simulink model "elevatorMod"  (R2020a)
settings: Solver=VariableStepAuto  StartTime=0.0  StopTime=inf  RelTol=1e-3
PreLoadFcn:
  | slplc.api.loadDataTypes;
undefined symbols (not defined in the file): BOOL, DINT, INT, slplc
libraries: simulink x1
(part 16 of 39)

== system elevatorMod/PLCControllerSuite/__Logic/Task/Program/__Logic/SUB/RungOutOverride ==
  In1 : Inport
  AND : Logic  AllPortsSameDT=off  OutDataTypeStr=boolean
  BlockEnableRead : Subsystem  DisableCoverage=on  TreatAsAtomicUnit=on  mask{PLCLabelTag=_Block_Enable, PLCBlockType=BlockEnableRead}
      mask prompts: PLCLabelTag "Label Tag:"
      mask init:
      | block = gcb;
      | maskObj = Simulink.Mask.get(block);
      | maskObj.Display = sprintf('disp(''%s'');', PLCLabelTag);
      mask Help: web([docroot '/plccoder/ref/blockenableread' '.html']);
      mask DialogControl PLCBlockTitle Prompt: Block Enable Read
      mask Display: disp('_Block_Enable');
  VariableWriteEnableWrite : Subsystem  DisableCoverage=on  TreatAsAtomicUnit=on  mask{PLCLabelTag=_Variable_Write_Enable, PLCBlockType=VariableWriteEnableWrite}
      mask prompts: PLCLabelTag "Label Tag:"
      mask init:
      | block = gcb;
      | maskObj = Simulink.Mask.get(block);
      | maskObj.Display = sprintf('disp(''%s'');', PLCLabelTag);
      mask Help: web([docroot '/plccoder/ref/variablewriteenablewrite' '.html']);
      mask DialogControl PLCBlockTitle Prompt: Variable Write_Enable_Write
      mask Display: disp('_Variable_Write_Enable');
  Out1 : Outport  VectorParamsAs1DForOutWhenUnconnected=off
  wires:
  AND/1 -> VariableWriteEnableWrite/1(In1), Out1/1
  BlockEnableRead/1(Out1) -> AND/1
  In1/1 -> AND/2

== system elevatorMod/PLCControllerSuite/__Logic/Task/Program/__Logic/TON/BlockEnableRead ==
  __CoreLabelRead : Subsystem  Tag=CoreVarReadBlock  DisableCoverage=on  TreatAsAtomicUnit=on  mask{PLCBlockType=CoreLabelRead}
      mask init:
      | slplc.callbacks.initRoutineLabelRead(gcb);
      mask Help: web([docroot '/plccoder/ref/__corelabelread' '.html']);
      mask DialogControl PLCBlockTitle Prompt: Core Label Read
  Out1 : Outport  VectorParamsAs1DForOutWhenUnconnected=off
  wires:
  __CoreLabelRead/1(Out1) -> Out1/1

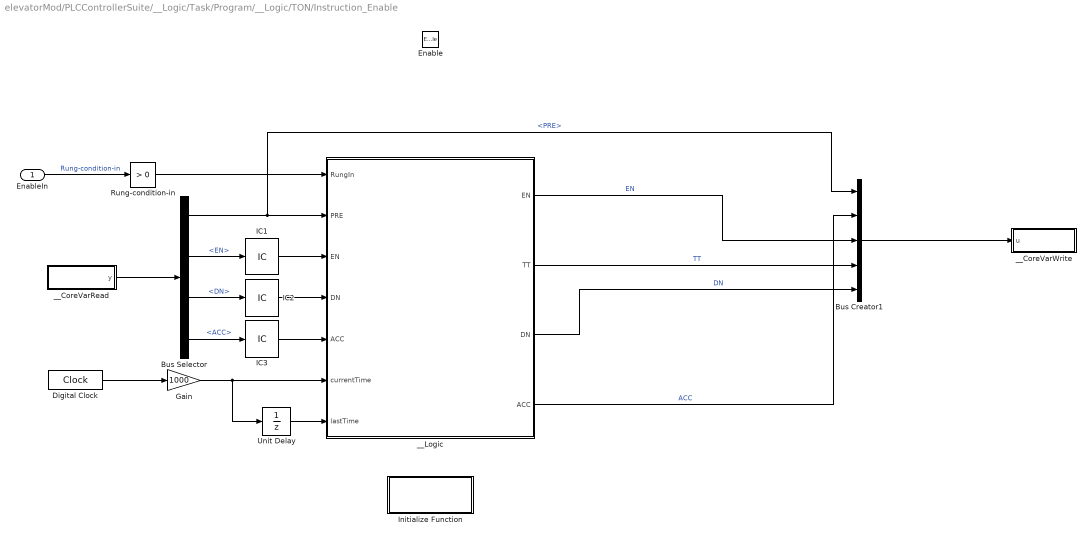
== system elevatorMod/PLCControllerSuite/__Logic/Task/Program/__Logic/TON/Instruction_Enable ==
  EnableIn : Inport
  Enable : EnablePort
  Bus Creator1 : BusCreator  Inputs=5  OutDataTypeStr=Bus: TIMER  NonVirtualBus=on
  Bus Selector : BusSelector  OutputSignals=PRE,EN,DN,ACC
  Digital Clock : DigitalClock  SampleTime=PLCTimerSampleTime
  Gain : Gain  Gain=1000
  IC1 : InitialCondition  Value=false
  IC2 : InitialCondition  Value=false
  IC3 : InitialCondition  Value=0
  Initialize Function : Subsystem  TreatAsAtomicUnit=on
  Rung-condition-in : simulink/Logic and Bit Operations/Compare To Zero  relop=>  OutDataTypeStr=boolean
  Unit Delay : UnitDelay  SampleTime=-1  HasFrameUpgradeWarning=on
  __CoreVarRead : Subsystem  Tag=CoreVarReadBlock  DisableCoverage=on  TreatAsAtomicUnit=on  mask{PLCBlockType=CoreVarRead}
      mask init:
      | slplc.callbacks.initCoreVariable(gcb, 'read');
      mask Help: web([docroot '/plccoder/ref/__corevarread' '.html']);
      mask DialogControl PLCBlockTitle Prompt: Core Variable Read
  __CoreVarWrite : Subsystem  Tag=CoreVarWriteBlock  DisableCoverage=on  TreatAsAtomicUnit=on  mask{PLCBlockType=CoreVarWrite}
      mask init:
      | slplc.callbacks.initCoreVariable(gcb, 'write');
      mask Help: web([docroot '/plccoder/ref/__corevarwrite' '.html']);
      mask DialogControl PLCBlockTitle Prompt: Core Variable Write
  __Logic : MATLAB Function  Priority=12  DisableCoverage=on
  wires:
  IC3/1 -> __Logic/5("ACC ")
  IC2/1 -> __Logic/4("DN ")
  IC1/1 -> __Logic/3("EN ")
  Rung-condition-in/1 -> __Logic/1(RungIn)
  Bus Selector/2 -> IC1/1  "<EN>"
  Gain/1 -> __Logic/6(currentTime), Unit Delay/1
  Bus Selector/3 -> IC2/1  "<DN>"
  __CoreVarRead/1(y) -> Bus Selector/1
  Unit Delay/1 -> __Logic/7(lastTime)
  Bus Creator1/1 -> __CoreVarWrite/1(u)
  __Logic/4(ACC) -> Bus Creator1/2  "ACC"
  __Logic/3(DN) -> Bus Creator1/5  "DN"
  Digital Clock/1 -> Gain/1
  EnableIn/1 -> Rung-condition-in/1  "Rung-condition-in"
  Bus Selector/1 -> Bus Creator1/1, __Logic/2(PRE)  "<PRE>"
  __Logic/2(TT) -> Bus Creator1/4  "TT"
  Bus Selector/4 -> IC3/1  "<ACC>"
  __Logic/1(EN) -> Bus Creator1/3  "EN"

== system elevatorMod/PLCControllerSuite/__Logic/Task/Program/__Logic/TON/RungInOverride ==
  In1 : Inport
  AND : Logic  AllPortsSameDT=off  OutDataTypeStr=boolean
  ForceRungInFalseRead : Subsystem  DisableCoverage=on  TreatAsAtomicUnit=on  mask{PLCLabelTag=_Force_RungIn_False, PLCBlockType=ForceRungInFalseRead}
      mask prompts: PLCLabelTag "Label Tag:"
      mask init:
      | block = gcb;
      | maskObj = Simulink.Mask.get(block);
      | maskObj.Display = sprintf('disp(''%s'');', PLCLabelTag);
      mask Help: web([docroot '/plccoder/ref/forcerunginfalseread' '.html']);
      mask DialogControl PLCBlockTitle Prompt: Force Rung-In False Read
      mask Display: disp('_Force_RungIn_False');
  NOT : Logic  Operator=NOT  IconShape=distinctive  AllPortsSameDT=off  OutDataTypeStr=boolean
  Out1 : Outport  VectorParamsAs1DForOutWhenUnconnected=off
  wires:
  AND/1 -> Out1/1
  In1/1 -> AND/2
  ForceRungInFalseRead/1(Out1) -> NOT/1
  NOT/1 -> AND/1

== system elevatorMod/PLCControllerSuite/__Logic/Task/Program/__Logic/TON/__CoreVarRead ==
  DataRead : DataStoreRead  DataStoreName=xxx_PLC_VAR_T
  y : Outport  VectorParamsAs1DForOutWhenUnconnected=off
  wires:
  DataRead/1 -> y/1

== system elevatorMod/PLCControllerSuite/__Logic/Task/Program/__Logic/Variable Read/__CoreVarRead ==
  DataRead : DataStoreRead  DataStoreName=xxx_PLC_VAR_VARVEL
  y : Outport  VectorParamsAs1DForOutWhenUnconnected=off
  wires:
  DataRead/1 -> y/1

== system elevatorMod/PLCControllerSuite/__Logic/Task/Program/__Logic/Variable Read1/__CoreVarRead ==
  DataRead : DataStoreRead  DataStoreName=xxx_PLC_VAR_Floor_1
  y : Outport  VectorParamsAs1DForOutWhenUnconnected=off
  wires:
  DataRead/1 -> y/1

== system elevatorMod/PLCControllerSuite/__Logic/Task/Program/__Logic/Variable Read10/__CoreVarRead ==
  DataRead : DataStoreRead  DataStoreName=xxx_PLC_VAR_VARVEL
  y : Outport  VectorParamsAs1DForOutWhenUnconnected=off
  wires:
  DataRead/1 -> y/1

== system elevatorMod/PLCControllerSuite/__Logic/Task/Program/__Logic/Variable Read11/__CoreVarRead ==
  DataRead : DataStoreRead  DataStoreName=xxx_PLC_VAR_VARVEL
  y : Outport  VectorParamsAs1DForOutWhenUnconnected=off
  wires:
  DataRead/1 -> y/1

== system elevatorMod/PLCControllerSuite/__Logic/Task/Program/__Logic/Variable Read12/__CoreVarRead ==
  DataRead : DataStoreRead  DataStoreName=xxx_PLC_VAR_VARVEL
  y : Outport  VectorParamsAs1DForOutWhenUnconnected=off
  wires:
  DataRead/1 -> y/1

== system elevatorMod/PLCControllerSuite/__Logic/Task/Program/__Logic/Variable Read13/__CoreVarRead ==
  DataRead : DataStoreRead  DataStoreName=xxx_PLC_VAR_VARVEL
  y : Outport  VectorParamsAs1DForOutWhenUnconnected=off
  wires:
  DataRead/1 -> y/1

== system elevatorMod/PLCControllerSuite/__Logic/Task/Program/__Logic/Variable Read14/__CoreVarRead ==
  DataRead : DataStoreRead  DataStoreName=xxx_PLC_VAR_VARVEL
  y : Outport  VectorParamsAs1DForOutWhenUnconnected=off
  wires:
  DataRead/1 -> y/1

== system elevatorMod/PLCControllerSuite/__Logic/Task/Program/__Logic/Variable Read15/__CoreVarRead ==
  DataRead : DataStoreRead  DataStoreName=xxx_PLC_VAR_VARVEL
  y : Outport  VectorParamsAs1DForOutWhenUnconnected=off
  wires:
  DataRead/1 -> y/1

== system elevatorMod/PLCControllerSuite/__Logic/Task/Program/__Logic/Variable Read16/__CoreVarRead ==
  DataRead : DataStoreRead  DataStoreName=xxx_PLC_VAR_Current_floor
  y : Outport  VectorParamsAs1DForOutWhenUnconnected=off
  wires:
  DataRead/1 -> y/1

== system elevatorMod/PLCControllerSuite/__Logic/Task/Program/__Logic/Variable Read2/__CoreVarRead ==
  DataRead : DataStoreRead  DataStoreName=xxx_PLC_VAR_Floor_2
  y : Outport  VectorParamsAs1DForOutWhenUnconnected=off
  wires:
  DataRead/1 -> y/1

== system elevatorMod/PLCControllerSuite/__Logic/Task/Program/__Logic/Variable Read3/__CoreVarRead ==
  DataRead : DataStoreRead  DataStoreName=xxx_PLC_VAR_Floor_3
  y : Outport  VectorParamsAs1DForOutWhenUnconnected=off
  wires:
  DataRead/1 -> y/1

== system elevatorMod/PLCControllerSuite/__Logic/Task/Program/__Logic/Variable Read4/__CoreVarRead ==
  DataRead : DataStoreRead  DataStoreName=xxx_PLC_VAR_Floor_1
  y : Outport  VectorParamsAs1DForOutWhenUnconnected=off
  wires:
  DataRead/1 -> y/1

== system elevatorMod/PLCControllerSuite/__Logic/Task/Program/__Logic/Variable Read5/__CoreVarRead ==
  DataRead : DataStoreRead  DataStoreName=xxx_PLC_VAR_Current_floor
  y : Outport  VectorParamsAs1DForOutWhenUnconnected=off
  wires:
  DataRead/1 -> y/1

== system elevatorMod/PLCControllerSuite/__Logic/Task/Program/__Logic/Variable Read6/__CoreVarRead ==
  DataRead : DataStoreRead  DataStoreName=xxx_PLC_VAR_Floor_2
  y : Outport  VectorParamsAs1DForOutWhenUnconnected=off
  wires:
  DataRead/1 -> y/1

== system elevatorMod/PLCControllerSuite/__Logic/Task/Program/__Logic/Variable Read7/__CoreVarRead ==
  DataRead : DataStoreRead  DataStoreName=xxx_PLC_VAR_Current_floor
  y : Outport  VectorParamsAs1DForOutWhenUnconnected=off
  wires:
  DataRead/1 -> y/1

== system elevatorMod/PLCControllerSuite/__Logic/Task/Program/__Logic/Variable Read8/__CoreVarRead ==
  DataRead : DataStoreRead  DataStoreName=xxx_PLC_VAR_Floor_3
  y : Outport  VectorParamsAs1DForOutWhenUnconnected=off
  wires:
  DataRead/1 -> y/1

== system elevatorMod/PLCControllerSuite/__Logic/Task/Program/__Logic/Variable Read9/__CoreVarRead ==
  DataRead : DataStoreRead  DataStoreName=xxx_PLC_VAR_Current_floor
  y : Outport  VectorParamsAs1DForOutWhenUnconnected=off
  wires:
  DataRead/1 -> y/1

== system elevatorMod/PLCControllerSuite/__Logic/Task/Program/__Logic/Variable Write1/VariableWriteEnableRead ==
  __CoreLabelRead : Subsystem  Tag=CoreVarReadBlock  DisableCoverage=on  TreatAsAtomicUnit=on  mask{PLCBlockType=CoreLabelRead}
      mask init:
      | slplc.callbacks.initRoutineLabelRead(gcb);
      mask Help: web([docroot '/plccoder/ref/__corelabelread' '.html']);
      mask DialogControl PLCBlockTitle Prompt: Core Label Read
  Out1 : Outport  VectorParamsAs1DForOutWhenUnconnected=off
  wires:
  __CoreLabelRead/1(Out1) -> Out1/1

== system elevatorMod/PLCControllerSuite/__Logic/Task/Program/__Logic/Variable Write1/__CoreVarRead ==
  DataRead : DataStoreRead  DataStoreName=xxx_PLC_VAR_Current_floor
  y : Outport  VectorParamsAs1DForOutWhenUnconnected=off
  wires:
  DataRead/1 -> y/1

== system elevatorMod/PLCControllerSuite/__Logic/Task/Program/__Logic/Variable Write1/__Enable ==
  VarIn : Inport
  Enable : EnablePort
  __CoreVarWrite : Subsystem  Tag=CoreVarWriteBlock  DisableCoverage=on  TreatAsAtomicUnit=on  mask{PLCBlockType=CoreVarWrite}
      mask init:
      | slplc.callbacks.initCoreVariable(gcb, 'write');
      mask Help: web([docroot '/plccoder/ref/__corevarwrite' '.html']);
      mask DialogControl PLCBlockTitle Prompt: Core Variable Write
  wires:
  VarIn/1 -> __CoreVarWrite/1(u)

== system elevatorMod/PLCControllerSuite/__Logic/Task/Program/__Logic/Variable Write2/VariableWriteEnableRead ==
  __CoreLabelRead : Subsystem  Tag=CoreVarReadBlock  DisableCoverage=on  TreatAsAtomicUnit=on  mask{PLCBlockType=CoreLabelRead}
      mask init:
      | slplc.callbacks.initRoutineLabelRead(gcb);
      mask Help: web([docroot '/plccoder/ref/__corelabelread' '.html']);
      mask DialogControl PLCBlockTitle Prompt: Core Label Read
  Out1 : Outport  VectorParamsAs1DForOutWhenUnconnected=off
  wires:
  __CoreLabelRead/1(Out1) -> Out1/1

== system elevatorMod/PLCControllerSuite/__Logic/Task/Program/__Logic/Variable Write2/__CoreVarRead ==
  DataRead : DataStoreRead  DataStoreName=xxx_PLC_VAR_Current_floor
  y : Outport  VectorParamsAs1DForOutWhenUnconnected=off
  wires:
  DataRead/1 -> y/1

== system elevatorMod/PLCControllerSuite/__Logic/Task/Program/__Logic/Variable Write2/__Enable ==
  VarIn : Inport
  Enable : EnablePort
  __CoreVarWrite : Subsystem  Tag=CoreVarWriteBlock  DisableCoverage=on  TreatAsAtomicUnit=on  mask{PLCBlockType=CoreVarWrite}
      mask init:
      | slplc.callbacks.initCoreVariable(gcb, 'write');
      mask Help: web([docroot '/plccoder/ref/__corevarwrite' '.html']);
      mask DialogControl PLCBlockTitle Prompt: Core Variable Write
  wires:
  VarIn/1 -> __CoreVarWrite/1(u)

== system elevatorMod/PLCControllerSuite/__Logic/Task/Program/__Logic/Variable Write3/VariableWriteEnableRead ==
  __CoreLabelRead : Subsystem  Tag=CoreVarReadBlock  DisableCoverage=on  TreatAsAtomicUnit=on  mask{PLCBlockType=CoreLabelRead}
      mask init:
      | slplc.callbacks.initRoutineLabelRead(gcb);
      mask Help: web([docroot '/plccoder/ref/__corelabelread' '.html']);
      mask DialogControl PLCBlockTitle Prompt: Core Label Read
  Out1 : Outport  VectorParamsAs1DForOutWhenUnconnected=off
  wires:
  __CoreLabelRead/1(Out1) -> Out1/1

== system elevatorMod/PLCControllerSuite/__Logic/Task/Program/__Logic/Variable Write3/__CoreVarRead ==
  DataRead : DataStoreRead  DataStoreName=xxx_PLC_VAR_Current_floor
  y : Outport  VectorParamsAs1DForOutWhenUnconnected=off
  wires:
  DataRead/1 -> y/1

== system elevatorMod/PLCControllerSuite/__Logic/Task/Program/__Logic/Variable Write3/__Enable ==
  VarIn : Inport
  Enable : EnablePort
  __CoreVarWrite : Subsystem  Tag=CoreVarWriteBlock  DisableCoverage=on  TreatAsAtomicUnit=on  mask{PLCBlockType=CoreVarWrite}
      mask init:
      | slplc.callbacks.initCoreVariable(gcb, 'write');
      mask Help: web([docroot '/plccoder/ref/__corevarwrite' '.html']);
      mask DialogControl PLCBlockTitle Prompt: Core Variable Write
  wires:
  VarIn/1 -> __CoreVarWrite/1(u)

== system elevatorMod/PLCControllerSuite/__Logic/Task/Program/__Logic/Variable Write4/VariableWriteEnableRead ==
  __CoreLabelRead : Subsystem  Tag=CoreVarReadBlock  DisableCoverage=on  TreatAsAtomicUnit=on  mask{PLCBlockType=CoreLabelRead}
      mask init:
      | slplc.callbacks.initRoutineLabelRead(gcb);
      mask Help: web([docroot '/plccoder/ref/__corelabelread' '.html']);
      mask DialogControl PLCBlockTitle Prompt: Core Label Read
  Out1 : Outport  VectorParamsAs1DForOutWhenUnconnected=off
  wires:
  __CoreLabelRead/1(Out1) -> Out1/1

== system elevatorMod/PLCControllerSuite/__Logic/Task/Program/__Logic/Variable Write4/__CoreVarRead ==
  DataRead : DataStoreRead  DataStoreName=xxx_PLC_VAR_VARVEL
  y : Outport  VectorParamsAs1DForOutWhenUnconnected=off
  wires:
  DataRead/1 -> y/1

== system elevatorMod/PLCControllerSuite/__Logic/Task/Program/__Logic/Variable Write4/__Enable ==
  VarIn : Inport
  Enable : EnablePort
  __CoreVarWrite : Subsystem  Tag=CoreVarWriteBlock  DisableCoverage=on  TreatAsAtomicUnit=on  mask{PLCBlockType=CoreVarWrite}
      mask init:
      | slplc.callbacks.initCoreVariable(gcb, 'write');
      mask Help: web([docroot '/plccoder/ref/__corevarwrite' '.html']);
      mask DialogControl PLCBlockTitle Prompt: Core Variable Write
  wires:
  VarIn/1 -> __CoreVarWrite/1(u)

== system elevatorMod/PLCControllerSuite/__Logic/Task/Program/__Logic/Variable Write5/VariableWriteEnableRead ==
  __CoreLabelRead : Subsystem  Tag=CoreVarReadBlock  DisableCoverage=on  TreatAsAtomicUnit=on  mask{PLCBlockType=CoreLabelRead}
      mask init:
      | slplc.callbacks.initRoutineLabelRead(gcb);
      mask Help: web([docroot '/plccoder/ref/__corelabelread' '.html']);
      mask DialogControl PLCBlockTitle Prompt: Core Label Read
  Out1 : Outport  VectorParamsAs1DForOutWhenUnconnected=off
  wires:
  __CoreLabelRead/1(Out1) -> Out1/1

== system elevatorMod/PLCControllerSuite/__Logic/Task/Program/__Logic/Variable Write5/__CoreVarRead ==
  DataRead : DataStoreRead  DataStoreName=xxx_PLC_VAR_VARVEL
  y : Outport  VectorParamsAs1DForOutWhenUnconnected=off
  wires:
  DataRead/1 -> y/1

== system elevatorMod/PLCControllerSuite/__Logic/Task/Program/__Logic/Variable Write5/__Enable ==
  VarIn : Inport
  Enable : EnablePort
  __CoreVarWrite : Subsystem  Tag=CoreVarWriteBlock  DisableCoverage=on  TreatAsAtomicUnit=on  mask{PLCBlockType=CoreVarWrite}
      mask init:
      | slplc.callbacks.initCoreVariable(gcb, 'write');
      mask Help: web([docroot '/plccoder/ref/__corevarwrite' '.html']);
      mask DialogControl PLCBlockTitle Prompt: Core Variable Write
  wires:
  VarIn/1 -> __CoreVarWrite/1(u)

== system elevatorMod/PLCControllerSuite/__Logic/Task/Program/__Logic/Variable Write6/VariableWriteEnableRead ==
  __CoreLabelRead : Subsystem  Tag=CoreVarReadBlock  DisableCoverage=on  TreatAsAtomicUnit=on  mask{PLCBlockType=CoreLabelRead}
      mask init:
      | slplc.callbacks.initRoutineLabelRead(gcb);
      mask Help: web([docroot '/plccoder/ref/__corelabelread' '.html']);
      mask DialogControl PLCBlockTitle Prompt: Core Label Read
  Out1 : Outport  VectorParamsAs1DForOutWhenUnconnected=off
  wires:
  __CoreLabelRead/1(Out1) -> Out1/1

== system elevatorMod/PLCControllerSuite/__Logic/Task/Program/__Logic/Variable Write6/__CoreVarRead ==
  DataRead : DataStoreRead  DataStoreName=xxx_PLC_VAR_VARVEL
  y : Outport  VectorParamsAs1DForOutWhenUnconnected=off
  wires:
  DataRead/1 -> y/1

== system elevatorMod/PLCControllerSuite/__Logic/Task/Program/__Logic/Variable Write6/__Enable ==
  VarIn : Inport
  Enable : EnablePort
  __CoreVarWrite : Subsystem  Tag=CoreVarWriteBlock  DisableCoverage=on  TreatAsAtomicUnit=on  mask{PLCBlockType=CoreVarWrite}
      mask init:
      | slplc.callbacks.initCoreVariable(gcb, 'write');
      mask Help: web([docroot '/plccoder/ref/__corevarwrite' '.html']);
      mask DialogControl PLCBlockTitle Prompt: Core Variable Write
  wires:
  VarIn/1 -> __CoreVarWrite/1(u)

== system elevatorMod/PLCControllerSuite/__Logic/Task/Program/__Logic/Variable Write7/VariableWriteEnableRead ==
  __CoreLabelRead : Subsystem  Tag=CoreVarReadBlock  DisableCoverage=on  TreatAsAtomicUnit=on  mask{PLCBlockType=CoreLabelRead}
      mask init:
      | slplc.callbacks.initRoutineLabelRead(gcb);
      mask Help: web([docroot '/plccoder/ref/__corelabelread' '.html']);
      mask DialogControl PLCBlockTitle Prompt: Core Label Read
  Out1 : Outport  VectorParamsAs1DForOutWhenUnconnected=off
  wires:
  __CoreLabelRead/1(Out1) -> Out1/1

== system elevatorMod/PLCControllerSuite/__Logic/Task/Program/__Logic/Variable Write7/__CoreVarRead ==
  DataRead : DataStoreRead  DataStoreName=xxx_PLC_VAR_VELOUT
  y : Outport  VectorParamsAs1DForOutWhenUnconnected=off
  wires:
  DataRead/1 -> y/1

== system elevatorMod/PLCControllerSuite/__Logic/Task/Program/__Logic/Variable Write7/__Enable ==
  VarIn : Inport
  Enable : EnablePort
  __CoreVarWrite : Subsystem  Tag=CoreVarWriteBlock  DisableCoverage=on  TreatAsAtomicUnit=on  mask{PLCBlockType=CoreVarWrite}
      mask init:
      | slplc.callbacks.initCoreVariable(gcb, 'write');
      mask Help: web([docroot '/plccoder/ref/__corevarwrite' '.html']);
      mask DialogControl PLCBlockTitle Prompt: Core Variable Write
  wires:
  VarIn/1 -> __CoreVarWrite/1(u)

== system elevatorMod/PLCControllerSuite/__Logic/Task/Program/__Logic/Variable Write8/VariableWriteEnableRead ==
  __CoreLabelRead : Subsystem  Tag=CoreVarReadBlock  DisableCoverage=on  TreatAsAtomicUnit=on  mask{PLCBlockType=CoreLabelRead}
      mask init:
      | slplc.callbacks.initRoutineLabelRead(gcb);
      mask Help: web([docroot '/plccoder/ref/__corelabelread' '.html']);
      mask DialogControl PLCBlockTitle Prompt: Core Label Read
  Out1 : Outport  VectorParamsAs1DForOutWhenUnconnected=off
  wires:
  __CoreLabelRead/1(Out1) -> Out1/1

== system elevatorMod/PLCControllerSuite/__Logic/Task/Program/__Logic/Variable Write8/__CoreVarRead ==
  DataRead : DataStoreRead  DataStoreName=xxx_PLC_VAR_FLOOROUT
  y : Outport  VectorParamsAs1DForOutWhenUnconnected=off
  wires:
  DataRead/1 -> y/1

== system elevatorMod/PLCControllerSuite/__Logic/Task/Program/__Logic/Variable Write8/__Enable ==
  VarIn : Inport
  Enable : EnablePort
  __CoreVarWrite : Subsystem  Tag=CoreVarWriteBlock  DisableCoverage=on  TreatAsAtomicUnit=on  mask{PLCBlockType=CoreVarWrite}
      mask init:
      | slplc.callbacks.initCoreVariable(gcb, 'write');
      mask Help: web([docroot '/plccoder/ref/__corevarwrite' '.html']);
      mask DialogControl PLCBlockTitle Prompt: Core Variable Write
  wires:
  VarIn/1 -> __CoreVarWrite/1(u)

== system elevatorMod/PLCControllerSuite/__Logic/Task/Program/__Logic/XIC/BlockEnableRead ==
  __CoreLabelRead : Subsystem  Tag=CoreVarReadBlock  DisableCoverage=on  TreatAsAtomicUnit=on  mask{PLCBlockType=CoreLabelRead}
      mask init:
      | slplc.callbacks.initRoutineLabelRead(gcb);
      mask Help: web([docroot '/plccoder/ref/__corelabelread' '.html']);
      mask DialogControl PLCBlockTitle Prompt: Core Label Read
  Out1 : Outport  VectorParamsAs1DForOutWhenUnconnected=off
  wires:
  __CoreLabelRead/1(Out1) -> Out1/1

== system elevatorMod/PLCControllerSuite/__Logic/Task/Program/__Logic/XIC/Instruction_Enable ==
  Rung-condition-in : Inport  OutDataTypeStr=BOOL
  Enable : EnablePort
  Logical Operator : Logic  OutDataTypeStr=BOOL
  __CoreVarRead : Subsystem  Tag=CoreVarReadBlock  DisableCoverage=on  TreatAsAtomicUnit=on  mask{PLCBlockType=CoreVarRead}
      mask init:
      | slplc.callbacks.initCoreVariable(gcb, 'read');
      mask Help: web([docroot '/plccoder/ref/__corevarread' '.html']);
      mask DialogControl PLCBlockTitle Prompt: Core Variable Read
  Rung-condition-out : Outport  VectorParamsAs1DForOutWhenUnconnected=off
  wires:
  __CoreVarRead/1(y) -> Logical Operator/2  "DataBit"
  Logical Operator/1 -> Rung-condition-out/1  "Rung-condition-out"
  Rung-condition-in/1 -> Logical Operator/1  "Rung-condition-in"

== system elevatorMod/PLCControllerSuite/__Logic/Task/Program/__Logic/XIC/RungInOverride ==
  In1 : Inport
  AND : Logic  AllPortsSameDT=off  OutDataTypeStr=boolean
  ForceRungInFalseRead : Subsystem  DisableCoverage=on  TreatAsAtomicUnit=on  mask{PLCLabelTag=_Force_RungIn_False, PLCBlockType=ForceRungInFalseRead}
      mask prompts: PLCLabelTag "Label Tag:"
      mask init:
      | block = gcb;
      | maskObj = Simulink.Mask.get(block);
      | maskObj.Display = sprintf('disp(''%s'');', PLCLabelTag);
      mask Help: web([docroot '/plccoder/ref/forcerunginfalseread' '.html']);
      mask DialogControl PLCBlockTitle Prompt: Force Rung-In False Read
      mask Display: disp('_Force_RungIn_False');
  NOT : Logic  Operator=NOT  IconShape=distinctive  AllPortsSameDT=off  OutDataTypeStr=boolean
  Out1 : Outport  VectorParamsAs1DForOutWhenUnconnected=off
  wires:
  NOT/1 -> AND/1
  ForceRungInFalseRead/1(Out1) -> NOT/1
  In1/1 -> AND/2
  AND/1 -> Out1/1

== system elevatorMod/PLCControllerSuite/__Logic/Task/Program/__Logic/XIC/__CoreVarRead ==
  DataRead : DataStoreRead  DataStoreName=xxx_PLC_VAR_Start
  y : Outport  VectorParamsAs1DForOutWhenUnconnected=off
  wires:
  DataRead/1 -> y/1

== system elevatorMod/PLCControllerSuite/__Logic/Task/Program/__Logic/XIC1/BlockEnableRead ==
  __CoreLabelRead : Subsystem  Tag=CoreVarReadBlock  DisableCoverage=on  TreatAsAtomicUnit=on  mask{PLCBlockType=CoreLabelRead}
      mask init:
      | slplc.callbacks.initRoutineLabelRead(gcb);
      mask Help: web([docroot '/plccoder/ref/__corelabelread' '.html']);
      mask DialogControl PLCBlockTitle Prompt: Core Label Read
  Out1 : Outport  VectorParamsAs1DForOutWhenUnconnected=off
  wires:
  __CoreLabelRead/1(Out1) -> Out1/1

== system elevatorMod/PLCControllerSuite/__Logic/Task/Program/__Logic/XIC1/Instruction_Enable ==
  Rung-condition-in : Inport  OutDataTypeStr=BOOL
  Enable : EnablePort
  Logical Operator : Logic  OutDataTypeStr=BOOL
  __CoreVarRead : Subsystem  Tag=CoreVarReadBlock  DisableCoverage=on  TreatAsAtomicUnit=on  mask{PLCBlockType=CoreVarRead}
      mask init:
      | slplc.callbacks.initCoreVariable(gcb, 'read');
      mask Help: web([docroot '/plccoder/ref/__corevarread' '.html']);
      mask DialogControl PLCBlockTitle Prompt: Core Variable Read
  Rung-condition-out : Outport  VectorParamsAs1DForOutWhenUnconnected=off
  wires:
  __CoreVarRead/1(y) -> Logical Operator/2  "DataBit"
  Logical Operator/1 -> Rung-condition-out/1  "Rung-condition-out"
  Rung-condition-in/1 -> Logical Operator/1  "Rung-condition-in"

== system elevatorMod/PLCControllerSuite/__Logic/Task/Program/__Logic/XIC1/RungInOverride ==
  In1 : Inport
  AND : Logic  AllPortsSameDT=off  OutDataTypeStr=boolean
  ForceRungInFalseRead : Subsystem  DisableCoverage=on  TreatAsAtomicUnit=on  mask{PLCLabelTag=_Force_RungIn_False, PLCBlockType=ForceRungInFalseRead}
      mask prompts: PLCLabelTag "Label Tag:"
      mask init:
      | block = gcb;
      | maskObj = Simulink.Mask.get(block);
      | maskObj.Display = sprintf('disp(''%s'');', PLCLabelTag);
      mask Help: web([docroot '/plccoder/ref/forcerunginfalseread' '.html']);
      mask DialogControl PLCBlockTitle Prompt: Force Rung-In False Read
      mask Display: disp('_Force_RungIn_False');
  NOT : Logic  Operator=NOT  IconShape=distinctive  AllPortsSameDT=off  OutDataTypeStr=boolean
  Out1 : Outport  VectorParamsAs1DForOutWhenUnconnected=off
  wires:
  NOT/1 -> AND/1
  ForceRungInFalseRead/1(Out1) -> NOT/1
  In1/1 -> AND/2
  AND/1 -> Out1/1

== system elevatorMod/PLCControllerSuite/__Logic/Task/Program/__Logic/XIC1/__CoreVarRead ==
  DataRead : DataStoreRead  DataStoreName=xxx_PLC_VAR_StartHold
  y : Outport  VectorParamsAs1DForOutWhenUnconnected=off
  wires:
  DataRead/1 -> y/1

== system elevatorMod/PLCControllerSuite/__Logic/Task/Program/__Logic/XIC10/BlockEnableRead ==
  __CoreLabelRead : Subsystem  Tag=CoreVarReadBlock  DisableCoverage=on  TreatAsAtomicUnit=on  mask{PLCBlockType=CoreLabelRead}
      mask init:
      | slplc.callbacks.initRoutineLabelRead(gcb);
      mask Help: web([docroot '/plccoder/ref/__corelabelread' '.html']);
      mask DialogControl PLCBlockTitle Prompt: Core Label Read
  Out1 : Outport  VectorParamsAs1DForOutWhenUnconnected=off
  wires:
  __CoreLabelRead/1(Out1) -> Out1/1

== system elevatorMod/PLCControllerSuite/__Logic/Task/Program/__Logic/XIC10/Instruction_Enable ==
  Rung-condition-in : Inport  OutDataTypeStr=BOOL
  Enable : EnablePort
  Logical Operator : Logic  OutDataTypeStr=BOOL
  __CoreVarRead : Subsystem  Tag=CoreVarReadBlock  DisableCoverage=on  TreatAsAtomicUnit=on  mask{PLCBlockType=CoreVarRead}
      mask init:
      | slplc.callbacks.initCoreVariable(gcb, 'read');
      mask Help: web([docroot '/plccoder/ref/__corevarread' '.html']);
      mask DialogControl PLCBlockTitle Prompt: Core Variable Read
  Rung-condition-out : Outport  VectorParamsAs1DForOutWhenUnconnected=off
  wires:
  Rung-condition-in/1 -> Logical Operator/1  "Rung-condition-in"
  Logical Operator/1 -> Rung-condition-out/1  "Rung-condition-out"
  __CoreVarRead/1(y) -> Logical Operator/2  "DataBit"

== system elevatorMod/PLCControllerSuite/__Logic/Task/Program/__Logic/XIC10/RungInOverride ==
  In1 : Inport
  AND : Logic  AllPortsSameDT=off  OutDataTypeStr=boolean
  ForceRungInFalseRead : Subsystem  DisableCoverage=on  TreatAsAtomicUnit=on  mask{PLCLabelTag=_Force_RungIn_False, PLCBlockType=ForceRungInFalseRead}
      mask prompts: PLCLabelTag "Label Tag:"
      mask init:
      | block = gcb;
      | maskObj = Simulink.Mask.get(block);
      | maskObj.Display = sprintf('disp(''%s'');', PLCLabelTag);
      mask Help: web([docroot '/plccoder/ref/forcerunginfalseread' '.html']);
      mask DialogControl PLCBlockTitle Prompt: Force Rung-In False Read
      mask Display: disp('_Force_RungIn_False');
  NOT : Logic  Operator=NOT  IconShape=distinctive  AllPortsSameDT=off  OutDataTypeStr=boolean
  Out1 : Outport  VectorParamsAs1DForOutWhenUnconnected=off
  wires:
  AND/1 -> Out1/1
  In1/1 -> AND/2
  ForceRungInFalseRead/1(Out1) -> NOT/1
  NOT/1 -> AND/1

== system elevatorMod/PLCControllerSuite/__Logic/Task/Program/__Logic/XIC10/__CoreVarRead ==
  DataRead : DataStoreRead  DataStoreName=xxx_PLC_VAR_StartHold
  y : Outport  VectorParamsAs1DForOutWhenUnconnected=off
  wires:
  DataRead/1 -> y/1

== system elevatorMod/PLCControllerSuite/__Logic/Task/Program/__Logic/XIC100/BlockEnableRead ==
  __CoreLabelRead : Subsystem  Tag=CoreVarReadBlock  DisableCoverage=on  TreatAsAtomicUnit=on  mask{PLCBlockType=CoreLabelRead}
      mask init:
      | slplc.callbacks.initRoutineLabelRead(gcb);
      mask Help: web([docroot '/plccoder/ref/__corelabelread' '.html']);
      mask DialogControl PLCBlockTitle Prompt: Core Label Read
  Out1 : Outport  VectorParamsAs1DForOutWhenUnconnected=off
  wires:
  __CoreLabelRead/1(Out1) -> Out1/1

== system elevatorMod/PLCControllerSuite/__Logic/Task/Program/__Logic/XIC100/Instruction_Enable ==
  Rung-condition-in : Inport  OutDataTypeStr=BOOL
  Enable : EnablePort
  Logical Operator : Logic  OutDataTypeStr=BOOL
  __CoreVarRead : Subsystem  Tag=CoreVarReadBlock  DisableCoverage=on  TreatAsAtomicUnit=on  mask{PLCBlockType=CoreVarRead}
      mask init:
      | slplc.callbacks.initCoreVariable(gcb, 'read');
      mask Help: web([docroot '/plccoder/ref/__corevarread' '.html']);
      mask DialogControl PLCBlockTitle Prompt: Core Variable Read
  Rung-condition-out : Outport  VectorParamsAs1DForOutWhenUnconnected=off
  wires:
  Rung-condition-in/1 -> Logical Operator/1  "Rung-condition-in"
  Logical Operator/1 -> Rung-condition-out/1  "Rung-condition-out"
  __CoreVarRead/1(y) -> Logical Operator/2  "DataBit"

== system elevatorMod/PLCControllerSuite/__Logic/Task/Program/__Logic/XIC100/RungInOverride ==
  In1 : Inport
  AND : Logic  AllPortsSameDT=off  OutDataTypeStr=boolean
  ForceRungInFalseRead : Subsystem  DisableCoverage=on  TreatAsAtomicUnit=on  mask{PLCLabelTag=_Force_RungIn_False, PLCBlockType=ForceRungInFalseRead}
      mask prompts: PLCLabelTag "Label Tag:"
      mask init:
      | block = gcb;
      | maskObj = Simulink.Mask.get(block);
      | maskObj.Display = sprintf('disp(''%s'');', PLCLabelTag);
      mask Help: web([docroot '/plccoder/ref/forcerunginfalseread' '.html']);
      mask DialogControl PLCBlockTitle Prompt: Force Rung-In False Read
      mask Display: disp('_Force_RungIn_False');
  NOT : Logic  Operator=NOT  IconShape=distinctive  AllPortsSameDT=off  OutDataTypeStr=boolean
  Out1 : Outport  VectorParamsAs1DForOutWhenUnconnected=off
  wires:
  AND/1 -> Out1/1
  In1/1 -> AND/2
  ForceRungInFalseRead/1(Out1) -> NOT/1
  NOT/1 -> AND/1

== system elevatorMod/PLCControllerSuite/__Logic/Task/Program/__Logic/XIC100/__CoreVarRead ==
  DataRead : DataStoreRead  DataStoreName=xxx_PLC_VAR_GOINGDN
  y : Outport  VectorParamsAs1DForOutWhenUnconnected=off
  wires:
  DataRead/1 -> y/1

== system elevatorMod/PLCControllerSuite/__Logic/Task/Program/__Logic/XIC101/BlockEnableRead ==
  __CoreLabelRead : Subsystem  Tag=CoreVarReadBlock  DisableCoverage=on  TreatAsAtomicUnit=on  mask{PLCBlockType=CoreLabelRead}
      mask init:
      | slplc.callbacks.initRoutineLabelRead(gcb);
      mask Help: web([docroot '/plccoder/ref/__corelabelread' '.html']);
      mask DialogControl PLCBlockTitle Prompt: Core Label Read
  Out1 : Outport  VectorParamsAs1DForOutWhenUnconnected=off
  wires:
  __CoreLabelRead/1(Out1) -> Out1/1

== system elevatorMod/PLCControllerSuite/__Logic/Task/Program/__Logic/XIC101/Instruction_Enable ==
  Rung-condition-in : Inport  OutDataTypeStr=BOOL
  Enable : EnablePort
  Logical Operator : Logic  OutDataTypeStr=BOOL
  __CoreVarRead : Subsystem  Tag=CoreVarReadBlock  DisableCoverage=on  TreatAsAtomicUnit=on  mask{PLCBlockType=CoreVarRead}
      mask init:
      | slplc.callbacks.initCoreVariable(gcb, 'read');
      mask Help: web([docroot '/plccoder/ref/__corevarread' '.html']);
      mask DialogControl PLCBlockTitle Prompt: Core Variable Read
  Rung-condition-out : Outport  VectorParamsAs1DForOutWhenUnconnected=off
  wires:
  __CoreVarRead/1(y) -> Logical Operator/2  "DataBit"
  Logical Operator/1 -> Rung-condition-out/1  "Rung-condition-out"
  Rung-condition-in/1 -> Logical Operator/1  "Rung-condition-in"

== system elevatorMod/PLCControllerSuite/__Logic/Task/Program/__Logic/XIC101/RungInOverride ==
  In1 : Inport
  AND : Logic  AllPortsSameDT=off  OutDataTypeStr=boolean
  ForceRungInFalseRead : Subsystem  DisableCoverage=on  TreatAsAtomicUnit=on  mask{PLCLabelTag=_Force_RungIn_False, PLCBlockType=ForceRungInFalseRead}
      mask prompts: PLCLabelTag "Label Tag:"
      mask init:
      | block = gcb;
      | maskObj = Simulink.Mask.get(block);
      | maskObj.Display = sprintf('disp(''%s'');', PLCLabelTag);
      mask Help: web([docroot '/plccoder/ref/forcerunginfalseread' '.html']);
      mask DialogControl PLCBlockTitle Prompt: Force Rung-In False Read
      mask Display: disp('_Force_RungIn_False');
  NOT : Logic  Operator=NOT  IconShape=distinctive  AllPortsSameDT=off  OutDataTypeStr=boolean
  Out1 : Outport  VectorParamsAs1DForOutWhenUnconnected=off
  wires:
  NOT/1 -> AND/1
  ForceRungInFalseRead/1(Out1) -> NOT/1
  In1/1 -> AND/2
  AND/1 -> Out1/1

== system elevatorMod/PLCControllerSuite/__Logic/Task/Program/__Logic/XIC101/__CoreVarRead ==
  DataRead : DataStoreRead  DataStoreName=xxx_PLC_VAR_StartHold
  y : Outport  VectorParamsAs1DForOutWhenUnconnected=off
  wires:
  DataRead/1 -> y/1

== system elevatorMod/PLCControllerSuite/__Logic/Task/Program/__Logic/XIC102/BlockEnableRead ==
  __CoreLabelRead : Subsystem  Tag=CoreVarReadBlock  DisableCoverage=on  TreatAsAtomicUnit=on  mask{PLCBlockType=CoreLabelRead}
      mask init:
      | slplc.callbacks.initRoutineLabelRead(gcb);
      mask Help: web([docroot '/plccoder/ref/__corelabelread' '.html']);
      mask DialogControl PLCBlockTitle Prompt: Core Label Read
  Out1 : Outport  VectorParamsAs1DForOutWhenUnconnected=off
  wires:
  __CoreLabelRead/1(Out1) -> Out1/1

== system elevatorMod/PLCControllerSuite/__Logic/Task/Program/__Logic/XIC102/Instruction_Enable ==
  Rung-condition-in : Inport  OutDataTypeStr=BOOL
  Enable : EnablePort
  Logical Operator : Logic  OutDataTypeStr=BOOL
  __CoreVarRead : Subsystem  Tag=CoreVarReadBlock  DisableCoverage=on  TreatAsAtomicUnit=on  mask{PLCBlockType=CoreVarRead}
      mask init:
      | slplc.callbacks.initCoreVariable(gcb, 'read');
      mask Help: web([docroot '/plccoder/ref/__corevarread' '.html']);
      mask DialogControl PLCBlockTitle Prompt: Core Variable Read
  Rung-condition-out : Outport  VectorParamsAs1DForOutWhenUnconnected=off
  wires:
  __CoreVarRead/1(y) -> Logical Operator/2  "DataBit"
  Logical Operator/1 -> Rung-condition-out/1  "Rung-condition-out"
  Rung-condition-in/1 -> Logical Operator/1  "Rung-condition-in"

== system elevatorMod/PLCControllerSuite/__Logic/Task/Program/__Logic/XIC102/RungInOverride ==
  In1 : Inport
  AND : Logic  AllPortsSameDT=off  OutDataTypeStr=boolean
  ForceRungInFalseRead : Subsystem  DisableCoverage=on  TreatAsAtomicUnit=on  mask{PLCLabelTag=_Force_RungIn_False, PLCBlockType=ForceRungInFalseRead}
      mask prompts: PLCLabelTag "Label Tag:"
      mask init:
      | block = gcb;
      | maskObj = Simulink.Mask.get(block);
      | maskObj.Display = sprintf('disp(''%s'');', PLCLabelTag);
      mask Help: web([docroot '/plccoder/ref/forcerunginfalseread' '.html']);
      mask DialogControl PLCBlockTitle Prompt: Force Rung-In False Read
      mask Display: disp('_Force_RungIn_False');
  NOT : Logic  Operator=NOT  IconShape=distinctive  AllPortsSameDT=off  OutDataTypeStr=boolean
  Out1 : Outport  VectorParamsAs1DForOutWhenUnconnected=off
  wires:
  NOT/1 -> AND/1
  ForceRungInFalseRead/1(Out1) -> NOT/1
  In1/1 -> AND/2
  AND/1 -> Out1/1

== system elevatorMod/PLCControllerSuite/__Logic/Task/Program/__Logic/XIC102/__CoreVarRead ==
  DataRead : DataStoreRead  DataStoreName=xxx_PLC_VAR_StartHold
  y : Outport  VectorParamsAs1DForOutWhenUnconnected=off
  wires:
  DataRead/1 -> y/1

== system elevatorMod/PLCControllerSuite/__Logic/Task/Program/__Logic/XIC103/BlockEnableRead ==
  __CoreLabelRead : Subsystem  Tag=CoreVarReadBlock  DisableCoverage=on  TreatAsAtomicUnit=on  mask{PLCBlockType=CoreLabelRead}
      mask init:
      | slplc.callbacks.initRoutineLabelRead(gcb);
      mask Help: web([docroot '/plccoder/ref/__corelabelread' '.html']);
      mask DialogControl PLCBlockTitle Prompt: Core Label Read
  Out1 : Outport  VectorParamsAs1DForOutWhenUnconnected=off
  wires:
  __CoreLabelRead/1(Out1) -> Out1/1

== system elevatorMod/PLCControllerSuite/__Logic/Task/Program/__Logic/XIC103/Instruction_Enable ==
  Rung-condition-in : Inport  OutDataTypeStr=BOOL
  Enable : EnablePort
  Logical Operator : Logic  OutDataTypeStr=BOOL
  __CoreVarRead : Subsystem  Tag=CoreVarReadBlock  DisableCoverage=on  TreatAsAtomicUnit=on  mask{PLCBlockType=CoreVarRead}
      mask init:
      | slplc.callbacks.initCoreVariable(gcb, 'read');
      mask Help: web([docroot '/plccoder/ref/__corevarread' '.html']);
      mask DialogControl PLCBlockTitle Prompt: Core Variable Read
  Rung-condition-out : Outport  VectorParamsAs1DForOutWhenUnconnected=off
  wires:
  __CoreVarRead/1(y) -> Logical Operator/2  "DataBit"
  Logical Operator/1 -> Rung-condition-out/1  "Rung-condition-out"
  Rung-condition-in/1 -> Logical Operator/1  "Rung-condition-in"

== system elevatorMod/PLCControllerSuite/__Logic/Task/Program/__Logic/XIC103/RungInOverride ==
  In1 : Inport
  AND : Logic  AllPortsSameDT=off  OutDataTypeStr=boolean
  ForceRungInFalseRead : Subsystem  DisableCoverage=on  TreatAsAtomicUnit=on  mask{PLCLabelTag=_Force_RungIn_False, PLCBlockType=ForceRungInFalseRead}
      mask prompts: PLCLabelTag "Label Tag:"
      mask init:
      | block = gcb;
      | maskObj = Simulink.Mask.get(block);
      | maskObj.Display = sprintf('disp(''%s'');', PLCLabelTag);
      mask Help: web([docroot '/plccoder/ref/forcerunginfalseread' '.html']);
      mask DialogControl PLCBlockTitle Prompt: Force Rung-In False Read
      mask Display: disp('_Force_RungIn_False');
  NOT : Logic  Operator=NOT  IconShape=distinctive  AllPortsSameDT=off  OutDataTypeStr=boolean
  Out1 : Outport  VectorParamsAs1DForOutWhenUnconnected=off
  wires:
  NOT/1 -> AND/1
  ForceRungInFalseRead/1(Out1) -> NOT/1
  In1/1 -> AND/2
  AND/1 -> Out1/1

== system elevatorMod/PLCControllerSuite/__Logic/Task/Program/__Logic/XIC103/__CoreVarRead ==
  DataRead : DataStoreRead  DataStoreName=xxx_PLC_VAR_StartHold
  y : Outport  VectorParamsAs1DForOutWhenUnconnected=off
  wires:
  DataRead/1 -> y/1

== system elevatorMod/PLCControllerSuite/__Logic/Task/Program/__Logic/XIC104/BlockEnableRead ==
  __CoreLabelRead : Subsystem  Tag=CoreVarReadBlock  DisableCoverage=on  TreatAsAtomicUnit=on  mask{PLCBlockType=CoreLabelRead}
      mask init:
      | slplc.callbacks.initRoutineLabelRead(gcb);
      mask Help: web([docroot '/plccoder/ref/__corelabelread' '.html']);
      mask DialogControl PLCBlockTitle Prompt: Core Label Read
  Out1 : Outport  VectorParamsAs1DForOutWhenUnconnected=off
  wires:
  __CoreLabelRead/1(Out1) -> Out1/1

== system elevatorMod/PLCControllerSuite/__Logic/Task/Program/__Logic/XIC104/Instruction_Enable ==
  Rung-condition-in : Inport  OutDataTypeStr=BOOL
  Enable : EnablePort
  Logical Operator : Logic  OutDataTypeStr=BOOL
  __CoreVarRead : Subsystem  Tag=CoreVarReadBlock  DisableCoverage=on  TreatAsAtomicUnit=on  mask{PLCBlockType=CoreVarRead}
      mask init:
      | slplc.callbacks.initCoreVariable(gcb, 'read');
      mask Help: web([docroot '/plccoder/ref/__corevarread' '.html']);
      mask DialogControl PLCBlockTitle Prompt: Core Variable Read
  Rung-condition-out : Outport  VectorParamsAs1DForOutWhenUnconnected=off
  wires:
  Rung-condition-in/1 -> Logical Operator/1  "Rung-condition-in"
  Logical Operator/1 -> Rung-condition-out/1  "Rung-condition-out"
  __CoreVarRead/1(y) -> Logical Operator/2  "DataBit"

== system elevatorMod/PLCControllerSuite/__Logic/Task/Program/__Logic/XIC104/RungInOverride ==
  In1 : Inport
  AND : Logic  AllPortsSameDT=off  OutDataTypeStr=boolean
  ForceRungInFalseRead : Subsystem  DisableCoverage=on  TreatAsAtomicUnit=on  mask{PLCLabelTag=_Force_RungIn_False, PLCBlockType=ForceRungInFalseRead}
      mask prompts: PLCLabelTag "Label Tag:"
      mask init:
      | block = gcb;
      | maskObj = Simulink.Mask.get(block);
      | maskObj.Display = sprintf('disp(''%s'');', PLCLabelTag);
      mask Help: web([docroot '/plccoder/ref/forcerunginfalseread' '.html']);
      mask DialogControl PLCBlockTitle Prompt: Force Rung-In False Read
      mask Display: disp('_Force_RungIn_False');
  NOT : Logic  Operator=NOT  IconShape=distinctive  AllPortsSameDT=off  OutDataTypeStr=boolean
  Out1 : Outport  VectorParamsAs1DForOutWhenUnconnected=off
  wires:
  AND/1 -> Out1/1
  In1/1 -> AND/2
  ForceRungInFalseRead/1(Out1) -> NOT/1
  NOT/1 -> AND/1

== system elevatorMod/PLCControllerSuite/__Logic/Task/Program/__Logic/XIC104/__CoreVarRead ==
  DataRead : DataStoreRead  DataStoreName=xxx_PLC_VAR_RMPDN
  y : Outport  VectorParamsAs1DForOutWhenUnconnected=off
  wires:
  DataRead/1 -> y/1

== system elevatorMod/PLCControllerSuite/__Logic/Task/Program/__Logic/XIC105/BlockEnableRead ==
  __CoreLabelRead : Subsystem  Tag=CoreVarReadBlock  DisableCoverage=on  TreatAsAtomicUnit=on  mask{PLCBlockType=CoreLabelRead}
      mask init:
      | slplc.callbacks.initRoutineLabelRead(gcb);
      mask Help: web([docroot '/plccoder/ref/__corelabelread' '.html']);
      mask DialogControl PLCBlockTitle Prompt: Core Label Read
  Out1 : Outport  VectorParamsAs1DForOutWhenUnconnected=off
  wires:
  __CoreLabelRead/1(Out1) -> Out1/1

== system elevatorMod/PLCControllerSuite/__Logic/Task/Program/__Logic/XIC105/Instruction_Enable ==
  Rung-condition-in : Inport  OutDataTypeStr=BOOL
  Enable : EnablePort
  Logical Operator : Logic  OutDataTypeStr=BOOL
  __CoreVarRead : Subsystem  Tag=CoreVarReadBlock  DisableCoverage=on  TreatAsAtomicUnit=on  mask{PLCBlockType=CoreVarRead}
      mask init:
      | slplc.callbacks.initCoreVariable(gcb, 'read');
      mask Help: web([docroot '/plccoder/ref/__corevarread' '.html']);
      mask DialogControl PLCBlockTitle Prompt: Core Variable Read
  Rung-condition-out : Outport  VectorParamsAs1DForOutWhenUnconnected=off
  wires:
  Rung-condition-in/1 -> Logical Operator/1  "Rung-condition-in"
  Logical Operator/1 -> Rung-condition-out/1  "Rung-condition-out"
  __CoreVarRead/1(y) -> Logical Operator/2  "DataBit"

== system elevatorMod/PLCControllerSuite/__Logic/Task/Program/__Logic/XIC105/RungInOverride ==
  In1 : Inport
  AND : Logic  AllPortsSameDT=off  OutDataTypeStr=boolean
  ForceRungInFalseRead : Subsystem  DisableCoverage=on  TreatAsAtomicUnit=on  mask{PLCLabelTag=_Force_RungIn_False, PLCBlockType=ForceRungInFalseRead}
      mask prompts: PLCLabelTag "Label Tag:"
      mask init:
      | block = gcb;
      | maskObj = Simulink.Mask.get(block);
      | maskObj.Display = sprintf('disp(''%s'');', PLCLabelTag);
      mask Help: web([docroot '/plccoder/ref/forcerunginfalseread' '.html']);
      mask DialogControl PLCBlockTitle Prompt: Force Rung-In False Read
      mask Display: disp('_Force_RungIn_False');
  NOT : Logic  Operator=NOT  IconShape=distinctive  AllPortsSameDT=off  OutDataTypeStr=boolean
  Out1 : Outport  VectorParamsAs1DForOutWhenUnconnected=off
  wires:
  AND/1 -> Out1/1
  In1/1 -> AND/2
  ForceRungInFalseRead/1(Out1) -> NOT/1
  NOT/1 -> AND/1

== system elevatorMod/PLCControllerSuite/__Logic/Task/Program/__Logic/XIC105/__CoreVarRead ==
  DataRead : DataStoreRead  DataStoreName=xxx_PLC_VAR_StartHold
  y : Outport  VectorParamsAs1DForOutWhenUnconnected=off
  wires:
  DataRead/1 -> y/1

== system elevatorMod/PLCControllerSuite/__Logic/Task/Program/__Logic/XIC106/BlockEnableRead ==
  __CoreLabelRead : Subsystem  Tag=CoreVarReadBlock  DisableCoverage=on  TreatAsAtomicUnit=on  mask{PLCBlockType=CoreLabelRead}
      mask init:
      | slplc.callbacks.initRoutineLabelRead(gcb);
      mask Help: web([docroot '/plccoder/ref/__corelabelread' '.html']);
      mask DialogControl PLCBlockTitle Prompt: Core Label Read
  Out1 : Outport  VectorParamsAs1DForOutWhenUnconnected=off
  wires:
  __CoreLabelRead/1(Out1) -> Out1/1

== system elevatorMod/PLCControllerSuite/__Logic/Task/Program/__Logic/XIC106/Instruction_Enable ==
  Rung-condition-in : Inport  OutDataTypeStr=BOOL
  Enable : EnablePort
  Logical Operator : Logic  OutDataTypeStr=BOOL
  __CoreVarRead : Subsystem  Tag=CoreVarReadBlock  DisableCoverage=on  TreatAsAtomicUnit=on  mask{PLCBlockType=CoreVarRead}
      mask init:
      | slplc.callbacks.initCoreVariable(gcb, 'read');
      mask Help: web([docroot '/plccoder/ref/__corevarread' '.html']);
      mask DialogControl PLCBlockTitle Prompt: Core Variable Read
  Rung-condition-out : Outport  VectorParamsAs1DForOutWhenUnconnected=off
  wires:
  Rung-condition-in/1 -> Logical Operator/1  "Rung-condition-in"
  Logical Operator/1 -> Rung-condition-out/1  "Rung-condition-out"
  __CoreVarRead/1(y) -> Logical Operator/2  "DataBit"

== system elevatorMod/PLCControllerSuite/__Logic/Task/Program/__Logic/XIC106/RungInOverride ==
  In1 : Inport
  AND : Logic  AllPortsSameDT=off  OutDataTypeStr=boolean
  ForceRungInFalseRead : Subsystem  DisableCoverage=on  TreatAsAtomicUnit=on  mask{PLCLabelTag=_Force_RungIn_False, PLCBlockType=ForceRungInFalseRead}
      mask prompts: PLCLabelTag "Label Tag:"
      mask init:
      | block = gcb;
      | maskObj = Simulink.Mask.get(block);
      | maskObj.Display = sprintf('disp(''%s'');', PLCLabelTag);
      mask Help: web([docroot '/plccoder/ref/forcerunginfalseread' '.html']);
      mask DialogControl PLCBlockTitle Prompt: Force Rung-In False Read
      mask Display: disp('_Force_RungIn_False');
  NOT : Logic  Operator=NOT  IconShape=distinctive  AllPortsSameDT=off  OutDataTypeStr=boolean
  Out1 : Outport  VectorParamsAs1DForOutWhenUnconnected=off
  wires:
  AND/1 -> Out1/1
  In1/1 -> AND/2
  ForceRungInFalseRead/1(Out1) -> NOT/1
  NOT/1 -> AND/1

== system elevatorMod/PLCControllerSuite/__Logic/Task/Program/__Logic/XIC106/__CoreVarRead ==
  DataRead : DataStoreRead  DataStoreName=xxx_PLC_VAR_StartHold
  y : Outport  VectorParamsAs1DForOutWhenUnconnected=off
  wires:
  DataRead/1 -> y/1

== system elevatorMod/PLCControllerSuite/__Logic/Task/Program/__Logic/XIC107/BlockEnableRead ==
  __CoreLabelRead : Subsystem  Tag=CoreVarReadBlock  DisableCoverage=on  TreatAsAtomicUnit=on  mask{PLCBlockType=CoreLabelRead}
      mask init:
      | slplc.callbacks.initRoutineLabelRead(gcb);
      mask Help: web([docroot '/plccoder/ref/__corelabelread' '.html']);
      mask DialogControl PLCBlockTitle Prompt: Core Label Read
  Out1 : Outport  VectorParamsAs1DForOutWhenUnconnected=off
  wires:
  __CoreLabelRead/1(Out1) -> Out1/1

== system elevatorMod/PLCControllerSuite/__Logic/Task/Program/__Logic/XIC107/Instruction_Enable ==
  Rung-condition-in : Inport  OutDataTypeStr=BOOL
  Enable : EnablePort
  Logical Operator : Logic  OutDataTypeStr=BOOL
  __CoreVarRead : Subsystem  Tag=CoreVarReadBlock  DisableCoverage=on  TreatAsAtomicUnit=on  mask{PLCBlockType=CoreVarRead}
      mask init:
      | slplc.callbacks.initCoreVariable(gcb, 'read');
      mask Help: web([docroot '/plccoder/ref/__corevarread' '.html']);
      mask DialogControl PLCBlockTitle Prompt: Core Variable Read
  Rung-condition-out : Outport  VectorParamsAs1DForOutWhenUnconnected=off
  wires:
  Rung-condition-in/1 -> Logical Operator/1  "Rung-condition-in"
  Logical Operator/1 -> Rung-condition-out/1  "Rung-condition-out"
  __CoreVarRead/1(y) -> Logical Operator/2  "DataBit"

== system elevatorMod/PLCControllerSuite/__Logic/Task/Program/__Logic/XIC107/RungInOverride ==
  In1 : Inport
  AND : Logic  AllPortsSameDT=off  OutDataTypeStr=boolean
  ForceRungInFalseRead : Subsystem  DisableCoverage=on  TreatAsAtomicUnit=on  mask{PLCLabelTag=_Force_RungIn_False, PLCBlockType=ForceRungInFalseRead}
      mask prompts: PLCLabelTag "Label Tag:"
      mask init:
      | block = gcb;
      | maskObj = Simulink.Mask.get(block);
      | maskObj.Display = sprintf('disp(''%s'');', PLCLabelTag);
      mask Help: web([docroot '/plccoder/ref/forcerunginfalseread' '.html']);
      mask DialogControl PLCBlockTitle Prompt: Force Rung-In False Read
      mask Display: disp('_Force_RungIn_False');
  NOT : Logic  Operator=NOT  IconShape=distinctive  AllPortsSameDT=off  OutDataTypeStr=boolean
  Out1 : Outport  VectorParamsAs1DForOutWhenUnconnected=off
  wires:
  AND/1 -> Out1/1
  In1/1 -> AND/2
  ForceRungInFalseRead/1(Out1) -> NOT/1
  NOT/1 -> AND/1

== system elevatorMod/PLCControllerSuite/__Logic/Task/Program/__Logic/XIC107/__CoreVarRead ==
  DataRead : DataStoreRead  DataStoreName=xxx_PLC_VAR_MTRON
  y : Outport  VectorParamsAs1DForOutWhenUnconnected=off
  wires:
  DataRead/1 -> y/1

== system elevatorMod/PLCControllerSuite/__Logic/Task/Program/__Logic/XIC108/BlockEnableRead ==
  __CoreLabelRead : Subsystem  Tag=CoreVarReadBlock  DisableCoverage=on  TreatAsAtomicUnit=on  mask{PLCBlockType=CoreLabelRead}
      mask init:
      | slplc.callbacks.initRoutineLabelRead(gcb);
      mask Help: web([docroot '/plccoder/ref/__corelabelread' '.html']);
      mask DialogControl PLCBlockTitle Prompt: Core Label Read
  Out1 : Outport  VectorParamsAs1DForOutWhenUnconnected=off
  wires:
  __CoreLabelRead/1(Out1) -> Out1/1

== system elevatorMod/PLCControllerSuite/__Logic/Task/Program/__Logic/XIC108/Instruction_Enable ==
  Rung-condition-in : Inport  OutDataTypeStr=BOOL
  Enable : EnablePort
  Logical Operator : Logic  OutDataTypeStr=BOOL
  __CoreVarRead : Subsystem  Tag=CoreVarReadBlock  DisableCoverage=on  TreatAsAtomicUnit=on  mask{PLCBlockType=CoreVarRead}
      mask init:
      | slplc.callbacks.initCoreVariable(gcb, 'read');
      mask Help: web([docroot '/plccoder/ref/__corevarread' '.html']);
      mask DialogControl PLCBlockTitle Prompt: Core Variable Read
  Rung-condition-out : Outport  VectorParamsAs1DForOutWhenUnconnected=off
  wires:
  __CoreVarRead/1(y) -> Logical Operator/2  "DataBit"
  Logical Operator/1 -> Rung-condition-out/1  "Rung-condition-out"
  Rung-condition-in/1 -> Logical Operator/1  "Rung-condition-in"
